simulink model "asm_basis_s"  (R2024a)
settings: Solver=ode45  StartTime=0.0  StopTime=0.5  FixedStep=Ta  MaxStep=1e-5  RelTol=1e-3  EnableMultiTasking=on
values from neighbouring files (symbols this model uses):
  ASM_Lh = 0.404    [init_asm_basis.m]
  ASM_Lr = ASM_Lrsigma + ASM_Lh    (= 0.41305)    [init_asm_basis.m]
  ASM_Ls = ASM_Lssigma + ASM_Lh    (= 0.41305)    [init_asm_basis.m]
  ASM_p = 1    [init_asm_basis.m]
  ASM_PSI_RN = 0.98    [init_asm_basis.m]
  ASM_Rr = 1.6    [init_asm_basis.m]
  ASM_sigma = 1-ASM_Lh^2/(ASM_Ls*ASM_Lr)    (= 0.0433403047275)    [init_asm_basis.m]
  CC_KAW = 1/ASM_TN    (= 303.359547356)    [init_asm_basis.m]
  CC_KI = CC_KP/ASM_T1    [init_asm_basis.m]
  CC_KP = (ASM_T1)/(2*ASM_K*ASM_Tsigma)    [init_asm_basis.m]
  f_sw = 5e3    (= 5000)    [init_asm_basis.m]
  FC_KAW = 1/FC_TN    (= 3.87362304806)    [init_asm_basis.m]
  FC_KI = FC_KP/FC_T1    [init_asm_basis.m]
  FC_KP = (FC_T1)/(2*FC_K*FC_Tsigma)    [init_asm_basis.m]
  imax = 6    [init_asm_basis.m]
  n_N = 2895    [init_asm_basis.m]
  SC_KAW = 1/(SC_a^2*SC_T_sigma)    [init_asm_basis.m]
  SC_KI = SC_KP/(SC_a^2*SC_T_sigma)    [init_asm_basis.m]
  SC_KP = SC_T1/(SC_a*SC_K*SC_T_sigma)    [init_asm_basis.m]
  Ta = 1/fa    (= 0.0002)    [init_asm_basis.m]
  udc = 400*sqrt(2)    [init_asm_basis.m]
  umax = udc/sqrt(3)    [init_asm_basis.m]
undefined symbols (not defined in the file or in its folder): DiscIntNeverNeededParam, plecs, sigbuilder_block
libraries: plecslib_extras2 x1, spsabctodq0Lib x1
settings Model: Creator=mabo  LastModifiedBy=mi
settings SolverCC: AlgebraicLoopSolver=TrustRegion
settings DataIOCC: LimitDataPoints=on  SaveFormat=Array  SignalLoggingSaveFormat=ModelDataLogs  ReturnWorkspaceOutputs=off
settings OptimizationCC: ExpressionDepthLimit=2147483647  LifeSpan=inf
settings DebuggingCC: UnderspecifiedInitializationDetection=Classic  MergeDetectMultiDrivingBlocksExec=none  SolverPrmCheckMsg=warning  FcnCallInpInsideContextMsg=warning  UnconnectedInputMsg=warning  UnconnectedOutputMsg=warning  UnconnectedLineMsg=warning  StateNameClashWarn=warning  SFUnexpectedBacktrackingDiag=warning  SFNoUnconditionalDefaultTransitionDiag=warning  SFExecutionAtInitializationDiag=none  ArithmeticOperatorsInVariantConditions=warning
settings HardwareCC: ProdBitPerPointer=32  ProdBitPerSizeT=32  ProdBitPerPtrDiffT=32  ProdLargestAtomicFloat=None  ProdIntDivRoundTo=Undefined  ProdEndianess=Unspecified  ProdWordSize=32  ProdHWDeviceType=32-bit Generic
settings ModelReferenceCC: EnableRefExpFcnMdlSchedulingChecks=on  PropagateSignalLabelsOutOfModel=off
settings SFSimCC: SimUseLocalCustomCode=off  SimParseCustomCode=off  CustomCodeUndefinedFunction=UseInterfaceOnly
settings RTWCC: RTWUseLocalCustomCode=off  GPUComputeCapability=3.5  DLArmComputeVersion=19.05
settings CodeAppCC: StateflowObjectComments=on
settings GRTTargetCC: TargetLangStandard=C89/C90 (ANSI)  CombineOutputUpdateFcns=off  GRTInterface=on
settings ConfigComp: CovMetricSettings=dw  CovSaveCumulativeToWorkspaceVar=on  CovSaveSingleToWorkspaceVar=on  CovExternalEMLEnable=off  CovSFcnEnable=off

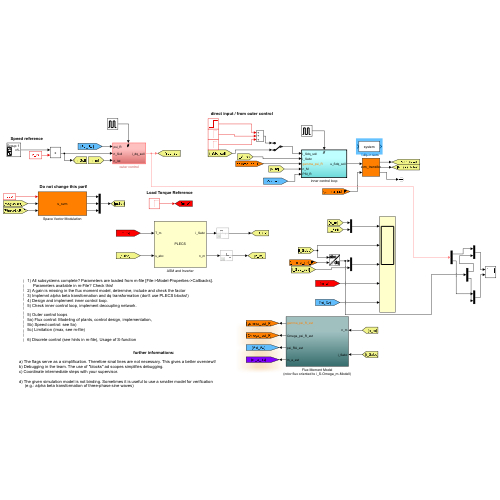
[thumbnail: Simulink's stored preview of the top-level diagram]
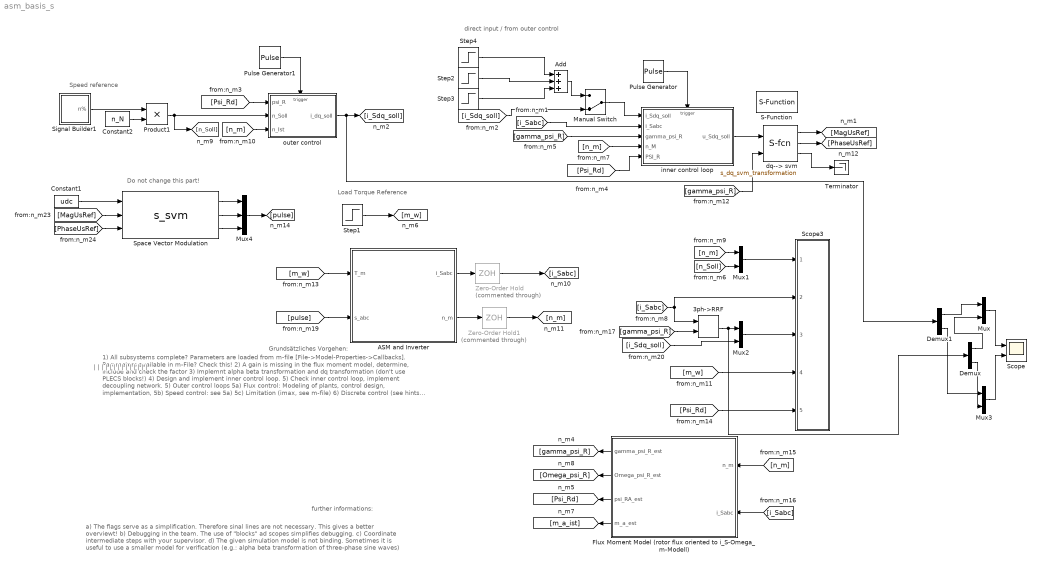
== system asm_basis_s ==
  note: Load Torque Reference
  note: Speed reference
  note: direct input / from outer control
  note: 1) All subsystems complete? Parameters are loaded from m-file [File->Model-Properties->Callbacks].
      |      Parameters available in m-File? Check this!
      | 2) A gain is missing in the flux moment model, determine, include and check the factor
      | 3) Implemnt alpha beta transformation and dq transformation (don't use PLECS blocks!)
      | 4) Design and implement inner control loop.
      | 5) Check inner control loop, implement decoupling network.
      |
      | 5) Outer control loops
      | 5a) Flux control: Modeling of plants, control design, implementation,
      | 5b) Speed control: see 5a)
      | 5c) Limitation (imax, see m-file)
      |
      | 6) Discrete control (see hints in m-file), Usage of S-function
  note: |
      | |
      | |
      | |
      | |
      | |
      | |
      | |
      | |
      | |
      | |
      | |
      | |
      | |
  note: Grundsätzliches Vorgehen:
  note: further informations:
  note: Do not change this part!
  note: a) The flags serve as a simplification. Therefore sinal lines are not necessary. This gives a better overviewt!
      | b) Debugging in the team. The use of "blocks" ad scopes simplifies debugging.
      | c) Coordinate intermediate steps with your supervisor.
      |
      | d) The given simulation model is not binding. Sometimes it is useful to use a smaller model for verification
      |      (e.g.: alpha beta transformation of three-phase sine waves)
  3ph->RRF : plecslib_extras2/Transformations/3ph->RRF
      settings: SourceProductName=PLECS Extras
  ASM and Inverter : Subsystem  LoadFcn=plecs('sl', 200);  InitFcn=plecs('sl', 214);  StartFcn=plecs('sl', 208);  StopFcn=plecs('sl', 209);  mask(PlecsCircuit){PLECSData=<binary blob, 7640 chars, not shown>}
      mask prompts: PLECSData "PLECS Data (Do not delete or modify!)"
      mask help: Drag this block into a Simulink model to create a new electrical circuit.
      mask init:
      | % PLACE CUSTOM INITIALIZATIONS ABOVE
      | % DO NOT REMOVE
      | plecs('sl', 215);
      | % DO NOT REMOVE
      settings: CopyFcn=plecs('sl', 203);  DeleteFcn=plecs('sl', 205);  UndoDeleteFcn=plecs('sl', 206);  PreSaveFcn=plecs('sl', 211);  PostSaveFcn=plecs('sl', 201);  NameChangeFcn=plecs('sl', 210);  DestroyFcn=plecs('sl', 207);  PreCopyFcn=plecs('sl', 216);  OpenFcn=plecs('sl', 202);  ErrorFcn=plerrorfcn
      mask Display: disp('PLECS')
  Add : Sum  Inputs=+++
  Constant1 : Constant  Value=udc
  Constant2 : Constant  Value=n_N
  Demux : Demux  Outputs=2
  Demux1 : Demux  Outputs=2
  Flux Moment Model (rotor flux oriented to i_S-Omega_m-Modell) : Subsystem
  Manual Switch : ManualSwitch  CurrentSetting=0
  Mux{,1..3} (4 alike) : Mux  Inputs=2
  Mux4 : Mux  Inputs=3
  Product1 : Product  RndMeth=Zero
  Pulse Generator : DiscretePulseGenerator  PulseType=Time based  Period=Ta  PulseWidth=5
  Pulse Generator1 : DiscretePulseGenerator  PulseType=Time based  Period=Ta  PulseWidth=5
  S-Function : S-Function  SFunctionDeploymentMode=off  EnableBusSupport=off
  Scope : Scope  NumInputPorts=2
  Scope3 : Subsystem  LoadFcn=plecs('sl', 300);  InitFcn=plecs('sl', 314);  StartFcn=plecs('sl', 308);  StopFcn=plecs('sl', 309);  mask{Settings=<binary blob, 2020 chars, not shown>}
      mask init:
      | plecsedit('sl', 315);
      settings: CopyFcn=plecs('sl', 303);  DeleteFcn=plecs('sl', 305);  UndoDeleteFcn=plecs('sl', 306);  PreSaveFcn=plecs('sl', 311);  NameChangeFcn=plecs('sl', 310);  DestroyFcn=plecs('sl', 307);  OpenFcn=plecs('sl', 302);  ErrorFcn=plerrorfcn
      mask Display: plot([0.1 0.9 0.9 0.1 0.1], [0.9 0.9 0.5 0.5 0.9])
  Signal Builder1 : Subsystem  Tag=STV Subsys  LoadFcn=sigbuilder_block('load');  StartFcn=sigbuilder_block('start');  StopFcn=sigbuilder_block('stop');  ClipboardFcn=sigbuilder_block('clipboard');  mask(Sigbuilder block){tuvar=[0:10]}
      mask help: Sigbuilder GUI
      mask init:
      | if ~strcmp(get_param(bdroot(gcbh),'SimulationStatus'),'stopped') tuvar = sigbuilder_block('maskInit'); end
      settings: CopyFcn=sigbuilder_block('copy');  DeleteFcn=sigbuilder_block('delete');  ModelCloseFcn=sigbuilder_block('modelClose');  PreSaveFcn=sigbuilder_block('preSave');  PauseFcn=sigbuilder_block('pause')  ContinueFcn=sigbuilder_block('continue')  NameChangeFcn=sigbuilder_block('namechange');  OpenFcn=sigbuilder_block('open',[29.25 172.2 550.5 395.55 ]);  CloseFcn=sigbuilder_block('close');
      mask Display: plot(0, 0, 100, 100,[2, 2, 32, 32, 2], [68, 8, 8, 68, 68],[32, 2], [38, 38], [32, 19, 2],[53, 60, 44], [32, 17, 17, 2],[16, 16, 31, 31]);txt = getActiveGroup(gcbh);text(2, 100, txt,'verticalAlignment', 'top');
  Space Vector Modulation : S-Function  FunctionName=s_svm  Parameters=f_sw*100,f_sw  SFunctionDeploymentMode=off  EnableBusSupport=off
  Step1 : Step  Time=9  After=2  SampleTime=0
  Step2 : Step  Time=0.1  Before=[1.5 0]  After=[1.5 2]  SampleTime=0
  Step3 : Step  Time=0.2  Before=[0 0]  After=[0 -2]  SampleTime=0
  Step4 : Step  Time=0.05  Before=[-1.5 0]  After=[0 0]  SampleTime=0
  Terminator : Terminator
  Zero-Order Hold : ZeroOrderHold  Commented=through  SampleTime=Ta
  Zero-Order Hold1 : ZeroOrderHold  Commented=through  SampleTime=Ta
  dq--> svm : S-Function  FunctionName=s_dq_svm_transformation  Parameters=f_sw  SFunctionDeploymentMode=off  EnableBusSupport=off
  inner control loop : Subsystem
  outer control : Subsystem
  wires:
  outer control/1(i_dq_soll) -> Demux1/1, [i_Sdq_soll]
  Step1/1 -> [m_w]
  [i_Sabc] -> inner control loop/2(i_Sabc)
  [i_Sdq_soll] -> Manual Switch/2
  [gamma_psi_R] -> inner control loop/3(gamma_psi_R)
  [n_m] -> outer control/3(n_Ist)
  Constant2/1 -> Product1/2
  Signal Builder1/1(n%) -> Product1/1
  Product1/1 -> [n_Soll], outer control/2(n_Soll)
  [m_w] -> ASM and Inverter/1(T_m)
  [pulse] -> ASM and Inverter/2(s_abc)
  Manual Switch/1 -> inner control loop/1(i_Sdq_soll)
  [Psi_Rd] -> outer control/1(psi_R)
  [Psi_Rd] -> inner control loop/5(PSI_R)
  [n_m] -> inner control loop/4(n_M)
  Add/1 -> Manual Switch/1
  Step2/1 -> Add/2
  Step3/1 -> Add/3
  Step4/1 -> Add/1
  ASM and Inverter/2(n_m) -> Zero-Order Hold1/1
  [n_m] -> Mux1/1
  [n_Soll] -> Mux1/2
  Mux1/1 -> Scope3/1(1)
  [i_Sabc] -> 3ph->RRF/1, Scope3/2(2)
  [gamma_psi_R] -> 3ph->RRF/2
  3ph->RRF/1 -> Demux/1, Mux2/1
  Mux2/1 -> Scope3/3(3)
  [m_w] -> Scope3/4(4)
  [Psi_Rd] -> Scope3/5(5)
  [PhaseUsRef] -> Space Vector Modulation/3
  [MagUsRef] -> Space Vector Modulation/2
  Constant1/1 -> Space Vector Modulation/1
  Space Vector Modulation/1 -> Mux4/1
  Space Vector Modulation/2 -> Mux4/2
  Space Vector Modulation/3 -> Mux4/3
  Mux4/1 -> [pulse]
  dq--> svm/1 -> [MagUsRef]
  dq--> svm/2 -> [PhaseUsRef]
  [gamma_psi_R] -> dq--> svm/2
  inner control loop/1(u_Sdq_soll) -> dq--> svm/1
  dq--> svm/3 -> Terminator/1
  [i_Sdq_soll] -> Mux2/2
  Flux Moment Model (rotor flux oriented to i_S-Omega_m-Modell)/1(gamma_psi_R_est) -> [gamma_psi_R]
  Flux Moment Model (rotor flux oriented to i_S-Omega_m-Modell)/4(m_a_est) -> [m_a_ist]
  [n_m] -> Flux Moment Model (rotor flux oriented to i_S-Omega_m-Modell)/1(n_m)
  [i_Sabc] -> Flux Moment Model (rotor flux oriented to i_S-Omega_m-Modell)/2(i_Sabc)
  Flux Moment Model (rotor flux oriented to i_S-Omega_m-Modell)/3(psi_RA_est) -> [Psi_Rd]
  Flux Moment Model (rotor flux oriented to i_S-Omega_m-Modell)/2(Omega_psi_R_est) -> [Omega_psi_R]
  Demux/1 -> Mux/2
  Demux1/1 -> Mux/1
  Mux/1 -> Scope/1
  Mux3/1 -> Scope/2
  Demux1/2 -> Mux3/1
  Demux/2 -> Mux3/2
  ASM and Inverter/1(i_Sabc) -> Zero-Order Hold/1
  Zero-Order Hold/1 -> [i_Sabc]
  Zero-Order Hold1/1 -> [n_m]
  Pulse Generator/1 -> inner control loop/Trigger
  Pulse Generator1/1 -> outer control/Trigger

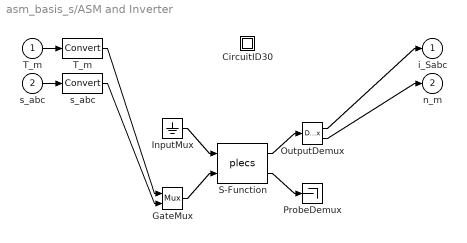
== system asm_basis_s/ASM and Inverter ==
  T_m : Inport  PortDimensions=1
  s_abc : Inport  Port=2  PortDimensions=3
  " CircuitID30 " : Subsystem
  " GateMux " : Mux  Inputs=[ 1 3 ]
  " InputMux " : Ground
  " OutputDemux " : Demux  Outputs=[ 3 1 ]
  " ProbeDemux " : Terminator
  " S-Function " : S-Function  FunctionName=plecs  SFunctionDeploymentMode=off  EnableBusSupport=off
  " T_m " : DataTypeConversion
  " s_abc " : DataTypeConversion
  i_Sabc : Outport  PortDimensions=3  VectorParamsAs1DForOutWhenUnconnected=off
  n_m : Outport  Port=2  PortDimensions=1  VectorParamsAs1DForOutWhenUnconnected=off
  wires:
  " InputMux "/1 -> " S-Function "/1
  " GateMux "/1 -> " S-Function "/2
  " S-Function "/1 -> " OutputDemux "/1
  " S-Function "/2 -> " ProbeDemux "/1
  T_m/1 -> " T_m "/1
  " T_m "/1 -> " GateMux "/1
  s_abc/1 -> " s_abc "/1
  " s_abc "/1 -> " GateMux "/2
  " OutputDemux "/1 -> i_Sabc/1
  " OutputDemux "/2 -> n_m/1

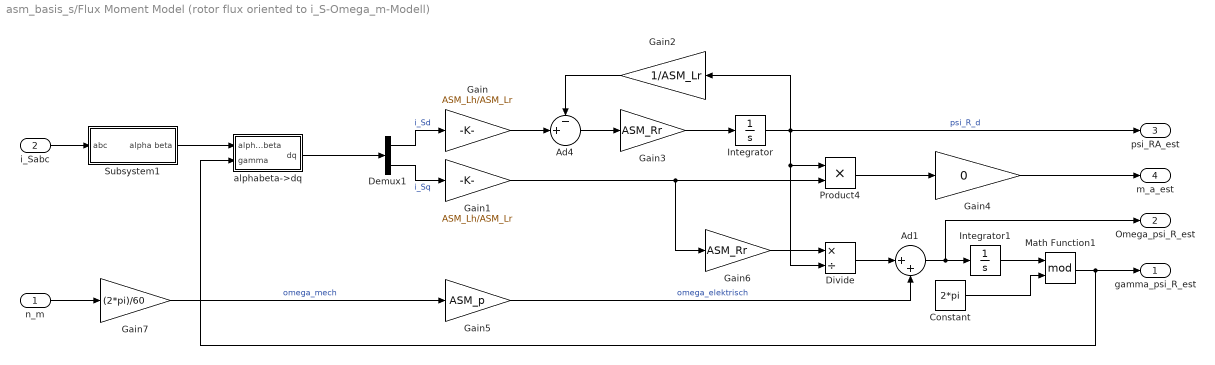
== system asm_basis_s/Flux Moment Model (rotor flux oriented to i_S-Omega_m-Modell) ==
  n_m : Inport
  i_Sabc : Inport  Port=2
  Ad1 : Sum  Inputs=|++
  Ad4 : Sum  Inputs=-+|
  Constant : Constant  Value=2*pi
  Demux1 : Demux  Outputs=2
  Divide : Product  Inputs=*/
  Gain : Gain  Gain=ASM_Lh/ASM_Lr
  Gain1 : Gain  Gain=ASM_Lh/ASM_Lr
  Gain2 : Gain  Gain=1/ASM_Lr
  Gain3 : Gain  Gain=ASM_Rr
  Gain4 : Gain  Gain=0
  Gain5 : Gain  Gain=ASM_p
  Gain6 : Gain  Gain=ASM_Rr
  Gain7 : Gain  Gain=(2*pi)/60
  Integrator : Integrator  InitialCondition=0.0001
  Integrator1 : Integrator  InitialCondition=0.0001
  Math Function1 : Math  Operator=mod  SignedPower=on
  Product4 : Product  RndMeth=Zero
  Subsystem1 : Subsystem
  alphabeta->dq : Subsystem
  gamma_psi_R_est : Outport  VectorParamsAs1DForOutWhenUnconnected=off
  Omega_psi_R_est : Outport  Port=2  VectorParamsAs1DForOutWhenUnconnected=off
  psi_RA_est : Outport  Port=3  VectorParamsAs1DForOutWhenUnconnected=off
  m_a_est : Outport  Port=4  VectorParamsAs1DForOutWhenUnconnected=off
  wires:
  Demux1/2 -> Gain1/1  "i_Sq"
  Demux1/1 -> Gain/1  "i_Sd"
  Gain/1 -> Ad4/2
  Ad4/1 -> Gain3/1
  Gain2/1 -> Ad4/1
  Gain3/1 -> Integrator/1
  Integrator/1 -> Gain2/1, psi_RA_est/1, Product4/1, Divide/2  "psi_R_d"
  Gain1/1 -> Product4/2, Gain6/1
  Product4/1 -> Gain4/1
  Gain4/1 -> m_a_est/1
  Divide/1 -> Ad1/1
  Ad1/1 -> Omega_psi_R_est/1, Integrator1/1
  Integrator1/1 -> Math Function1/1
  n_m/1 -> Gain7/1
  Gain5/1 -> Ad1/2  "omega_elektrisch"
  Math Function1/1 -> gamma_psi_R_est/1, alphabeta->dq/2(gamma)
  Gain6/1 -> Divide/1
  Subsystem1/1(alpha beta) -> alphabeta->dq/1(alphabeta)
  i_Sabc/1 -> Subsystem1/1(abc)
  alphabeta->dq/1(dq) -> Demux1/1
  Gain7/1 -> Gain5/1  "omega_mech"
  Constant/1 -> Math Function1/2

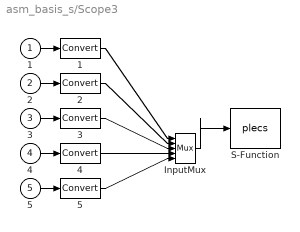
== system asm_basis_s/Scope3 ==
  1 : Inport
  2 : Inport  Port=2
  3 : Inport  Port=3
  4 : Inport  Port=4
  5 : Inport  Port=5
  " 1 " : DataTypeConversion
  " 2 " : DataTypeConversion
  " 3 " : DataTypeConversion
  " 4 " : DataTypeConversion
  " 5 " : DataTypeConversion
  " InputMux " : Mux  Inputs=5
  " S-Function " : S-Function  FunctionName=plecs  SFunctionDeploymentMode=off  EnableBusSupport=off
  wires:
  " InputMux "/1 -> " S-Function "/1
  1/1 -> " 1 "/1
  " 1 "/1 -> " InputMux "/1
  2/1 -> " 2 "/1
  " 2 "/1 -> " InputMux "/2
  3/1 -> " 3 "/1
  " 3 "/1 -> " InputMux "/3
  4/1 -> " 4 "/1
  " 4 "/1 -> " InputMux "/4
  5/1 -> " 5 "/1
  " 5 "/1 -> " InputMux "/5

== system asm_basis_s/Signal Builder1 ==
  Demux : Demux  Tag=STV Demux  Outputs=1
      settings: DisplayOption=none
  FromWs : FromWorkspace  Tag=STV FromWs  VariableName=tuvar
      SigBuilderData=|
      | common.afterFinalStr = 'Extrapolate'
      | common.sampleTime = 0
      | dataSet.timeRange = [0 1]
      | dataSet.name = 'Group 1'
      | sbobj.Groups.Name = 'Group 1'
      | sbobj.Groups.Signals.Name = 'n%'
      | sbobj.Groups.Signals.XData = [0 0.102 0.102 0.354 0.354 1]
      | sbobj.Groups.Signals.YData = [0 0 1 1 0.6 0.6]
      | sbobj.Groups.TimeRange = [0 1]
  n% : Outport  Tag=STV Outport  VectorParamsAs1DForOutWhenUnconnected=off
  wires:
  FromWs/1 -> Demux/1
  Demux/1 -> n%/1

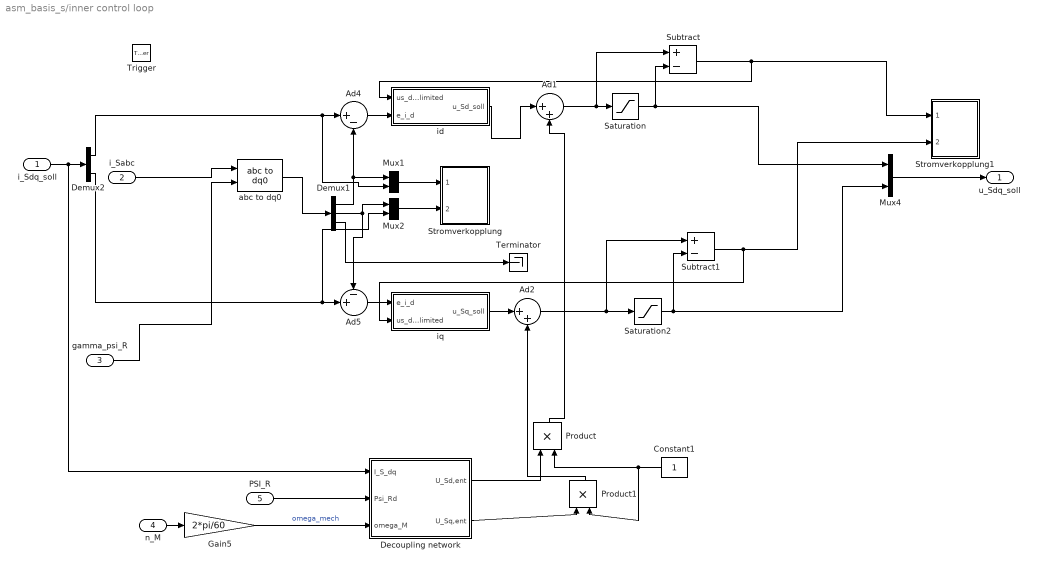
== system asm_basis_s/inner control loop ==
  i_Sdq_soll : Inport
  i_Sabc : Inport  Port=2
  gamma_psi_R : Inport  Port=3
  n_M : Inport  Port=4
  PSI_R : Inport  Port=5
  Trigger : TriggerPort  VariantControl=(inherit)  PortDimensions=1
  Ad1 : Sum  Inputs=|++
  Ad2 : Sum  Inputs=|++
  Ad4 : Sum  Inputs=|+-
  Ad5 : Sum  Inputs=-+|
  Constant1 : Constant
  Decoupling network : Subsystem
  Demux1 : Demux  Outputs=3
  Demux2 : Demux  Outputs=2
  Gain5 : Gain  Gain=2*pi/60
  Mux1 : Mux  Inputs=[1 1]
  Mux2 : Mux  Inputs=[1 1]
  Mux4 : Mux  Inputs=2
  Product : Product  RndMeth=Zero
  Product1 : Product  RndMeth=Zero
  Saturation : Saturate  UpperLimit=umax  LowerLimit=-umax
  Saturation2 : Saturate  UpperLimit=umax  LowerLimit=-umax
  Stromverkopplung : Subsystem  LoadFcn=plecs('sl', 300);  InitFcn=plecs('sl', 314);  StartFcn=plecs('sl', 308);  StopFcn=plecs('sl', 309);  mask{Settings=<binary blob, 1300 chars, not shown>}
      mask init:
      | plecsedit('sl', 315);
      settings: CopyFcn=plecs('sl', 303);  DeleteFcn=plecs('sl', 305);  UndoDeleteFcn=plecs('sl', 306);  PreSaveFcn=plecs('sl', 311);  NameChangeFcn=plecs('sl', 310);  DestroyFcn=plecs('sl', 307);  OpenFcn=plecs('sl', 302);  ErrorFcn=plerrorfcn
      mask Display: plot([0.1 0.9 0.9 0.1 0.1], [0.9 0.9 0.5 0.5 0.9])
  Stromverkopplung1 : Subsystem  LoadFcn=plecs('sl', 300);  InitFcn=plecs('sl', 314);  StartFcn=plecs('sl', 308);  StopFcn=plecs('sl', 309);  mask{Settings=<binary blob, 1192 chars, not shown>}
      mask init:
      | plecsedit('sl', 315);
      settings: CopyFcn=plecs('sl', 303);  DeleteFcn=plecs('sl', 305);  UndoDeleteFcn=plecs('sl', 306);  PreSaveFcn=plecs('sl', 311);  NameChangeFcn=plecs('sl', 310);  DestroyFcn=plecs('sl', 307);  OpenFcn=plecs('sl', 302);  ErrorFcn=plerrorfcn
      mask Display: plot([0.1 0.9 0.9 0.1 0.1], [0.9 0.9 0.5 0.5 0.9])
  Subtract : Sum  Inputs=+-
  Subtract1 : Sum  Inputs=+-
  Terminator : Terminator
  abc to dq0 : spsabctodq0Lib/abc to dq0  Alignment=Aligned with phase A axis
  id : Subsystem
  iq : Subsystem
  u_Sdq_soll : Outport  VectorParamsAs1DForOutWhenUnconnected=off
  wires:
  Ad4/1 -> id/2(e_i_d)
  Demux1/1 -> Ad4/2, Mux1/1
  Demux2/1 -> Ad4/1, Mux1/2
  Demux1/2 -> Ad5/1, Mux2/1
  Demux2/2 -> Mux2/2, Ad5/2
  Ad5/1 -> iq/1(e_i_d)
  i_Sdq_soll/1 -> Demux2/1, Decoupling network/1(I_S_dq)
  Mux1/1 -> Stromverkopplung/1(1)
  Mux2/1 -> Stromverkopplung/2(2)
  PSI_R/1 -> Decoupling network/2(Psi_Rd)
  n_M/1 -> Gain5/1
  Gain5/1 -> Decoupling network/3(omega_M)  "omega_mech"
  Decoupling network/2(U_Sq,ent) -> Product1/1
  Mux4/1 -> u_Sdq_soll/1
  Subtract1/1 -> iq/2(us_delta_limited), Stromverkopplung1/2(2)
  Constant1/1 -> Product/2, Product1/2
  Decoupling network/1(U_Sd,ent) -> Product/1
  Product/1 -> Ad1/2
  Product1/1 -> Ad2/2
  Demux1/3 -> Terminator/1
  Subtract/1 -> id/1(us_delta_limited), Stromverkopplung1/1(1)
  abc to dq0/1 -> Demux1/1
  Saturation/1 -> Mux4/1, Subtract/2
  id/1(u_Sd_soll) -> Ad1/1
  Saturation2/1 -> Mux4/2, Subtract1/2
  iq/1(u_Sq_soll) -> Ad2/1
  Ad1/1 -> Subtract/1, Saturation/1
  Ad2/1 -> Subtract1/1, Saturation2/1
  i_Sabc/1 -> abc to dq0/1
  gamma_psi_R/1 -> abc to dq0/2

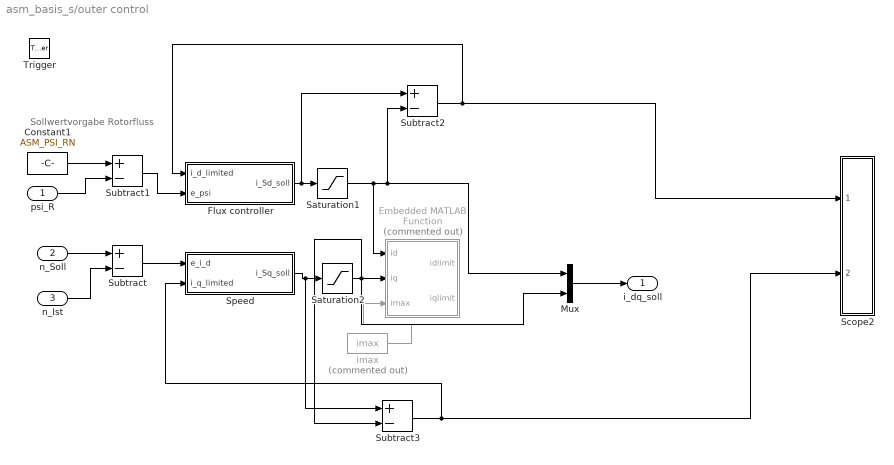
== system asm_basis_s/outer control ==
  note: Sollwertvorgabe
      |  Rotorfluss
  psi_R : Inport
  n_Soll : Inport  Port=2
  n_Ist : Inport  Port=3
  Trigger : TriggerPort  VariantControl=(inherit)  PortDimensions=1
  Constant1 : Constant  Value=ASM_PSI_RN
  Embedded MATLAB Function : MATLAB Function  Commented=on  TreatAsAtomicUnit=on
  Flux controller : Subsystem
  Mux : Mux  Inputs=[1 1]
  Saturation1 : Saturate  UpperLimit=imax  LowerLimit=-imax
  Saturation2 : Saturate  UpperLimit=imax  LowerLimit=-imax
  Scope2 : Subsystem  LoadFcn=plecs('sl', 300);  InitFcn=plecs('sl', 314);  StartFcn=plecs('sl', 308);  StopFcn=plecs('sl', 309);  mask{Settings=<binary blob, 1192 chars, not shown>}
      mask init:
      | plecsedit('sl', 315);
      settings: CopyFcn=plecs('sl', 303);  DeleteFcn=plecs('sl', 305);  UndoDeleteFcn=plecs('sl', 306);  PreSaveFcn=plecs('sl', 311);  NameChangeFcn=plecs('sl', 310);  DestroyFcn=plecs('sl', 307);  OpenFcn=plecs('sl', 302);  ErrorFcn=plerrorfcn
      mask Display: plot([0.1 0.9 0.9 0.1 0.1], [0.9 0.9 0.5 0.5 0.9])
  Speed : Subsystem
  Subtract{,1..3} (4 alike) : Sum  Inputs=+-
  imax : Constant  Commented=on  Value=imax
  i_dq_soll : Outport  InitialOutput=[0 0]  VectorParamsAs1DForOutWhenUnconnected=off
  wires:
  Flux controller/1(i_Sd_soll) -> Subtract2/1, Saturation1/1
  Speed/1(i_Sq_soll) -> Subtract3/1, Saturation2/1
  imax/1 -> Embedded MATLAB Function/3(imax)
  n_Soll/1 -> Subtract/1
  n_Ist/1 -> Subtract/2
  Subtract/1 -> Speed/1(e_i_d)
  Constant1/1 -> Subtract1/1
  psi_R/1 -> Subtract1/2
  Subtract1/1 -> Flux controller/2(e_psi)
  Mux/1 -> i_dq_soll/1
  Saturation1/1 -> Subtract2/2, Mux/1, Embedded MATLAB Function/1(id)
  Saturation2/1 -> Mux/2, Subtract3/2, Embedded MATLAB Function/2(iq)
  Subtract2/1 -> Flux controller/1(i_d_limited), Scope2/1(1)
  Subtract3/1 -> Speed/2(i_q_limited), Scope2/2(2)

== system asm_basis_s/ASM and Inverter/ CircuitID30  ==

== system asm_basis_s/Flux Moment Model (rotor flux oriented to i_S-Omega_m-Modell)/Subsystem1 ==
  note: Amplitudeninvariant
  abc : Inport  PortDimensions=3
  Mux : Mux  Inputs=2
  alpha : Fcn  Expr=(2*u(1)-u(2)-u(3))/3
  beta : Fcn  Expr=(u(2)-u(3))/sqrt(3)
  alpha beta : Outport  VectorParamsAs1DForOutWhenUnconnected=off
  wires:
  alpha/1 -> Mux/1
  beta/1 -> Mux/2
  abc/1 -> beta/1, alpha/1
  Mux/1 -> alpha beta/1

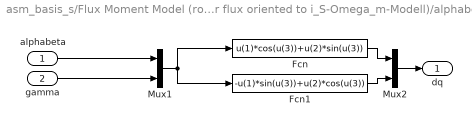
== system asm_basis_s/Flux Moment Model (rotor flux oriented to i_S-Omega_m-Modell)/alphabeta->dq ==
  alphabeta : Inport
  gamma : Inport  Port=2
  Fcn : Fcn  Expr=u(1)*cos(u(3))+u(2)*sin(u(3))
  Fcn1 : Fcn  Expr=-u(1)*sin(u(3))+u(2)*cos(u(3))
  Mux1 : Mux  Inputs=2
  Mux2 : Mux  Inputs=2
  dq : Outport  VectorParamsAs1DForOutWhenUnconnected=off
  wires:
  Mux2/1 -> dq/1
  Mux1/1 -> Fcn1/1, Fcn/1
  Fcn1/1 -> Mux2/2
  Fcn/1 -> Mux2/1
  alphabeta/1 -> Mux1/1
  gamma/1 -> Mux1/2

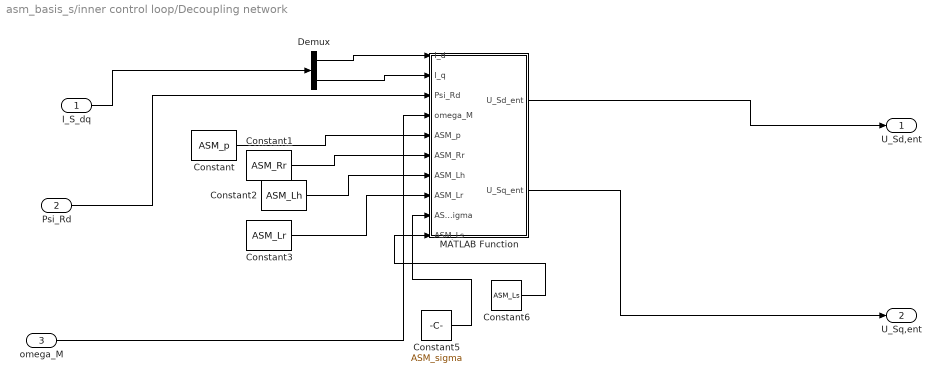
== system asm_basis_s/inner control loop/Decoupling network ==
  I_S_dq : Inport
  Psi_Rd : Inport  Port=2
  omega_M : Inport  Port=3
  Constant : Constant  Value=ASM_p
  Constant1 : Constant  Value=ASM_Rr
  Constant2 : Constant  Value=ASM_Lh
  Constant3 : Constant  Value=ASM_Lr
  Constant5 : Constant  Value=ASM_sigma
  Constant6 : Constant  Value=ASM_Ls
  Demux : Demux  Outputs=2
  MATLAB Function : MATLAB Function  TreatAsAtomicUnit=on
  U_Sd,ent : Outport  VectorParamsAs1DForOutWhenUnconnected=off
  U_Sq,ent : Outport  Port=2  VectorParamsAs1DForOutWhenUnconnected=off
  wires:
  I_S_dq/1 -> Demux/1
  Psi_Rd/1 -> MATLAB Function/3(Psi_Rd)
  omega_M/1 -> MATLAB Function/4(omega_M)
  MATLAB Function/1(U_Sd_ent) -> U_Sd,ent/1
  MATLAB Function/2(U_Sq_ent) -> U_Sq,ent/1
  Constant/1 -> MATLAB Function/5(ASM_p)
  Constant1/1 -> MATLAB Function/6(ASM_Rr)
  Constant2/1 -> MATLAB Function/7(ASM_Lh)
  Constant3/1 -> MATLAB Function/8(ASM_Lr)
  Demux/1 -> MATLAB Function/1(I_d)
  Demux/2 -> MATLAB Function/2(I_q)
  Constant5/1 -> MATLAB Function/9(ASM_sigma)
  Constant6/1 -> MATLAB Function/10(ASM_Ls)

== system asm_basis_s/inner control loop/Stromverkopplung ==
  1 : Inport
  2 : Inport  Port=2
  " InputMux " : Subsystem
      mask Display: disp('Mux')
  " S-Function " : S-Function  FunctionName=plecs  SFunctionDeploymentMode=off  EnableBusSupport=off
  wires:
  2/1 -> " InputMux "/2(In2)
  1/1 -> " InputMux "/1(In1)
  " InputMux "/1(Out) -> " S-Function "/1

== system asm_basis_s/inner control loop/Stromverkopplung1 ==
  1 : Inport
  2 : Inport  Port=2
  " InputMux " : Subsystem
      mask Display: disp('Mux')
  " S-Function " : S-Function  FunctionName=plecs  SFunctionDeploymentMode=off  EnableBusSupport=off
  wires:
  " InputMux "/1(Out) -> " S-Function "/1
  1/1 -> " InputMux "/1(In1)
  2/1 -> " InputMux "/2(In2)

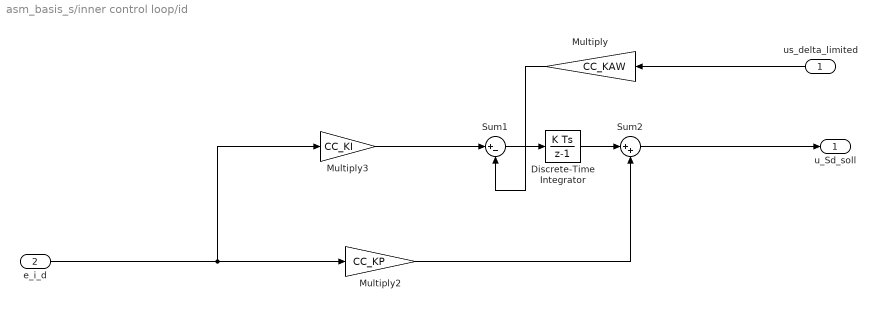
== system asm_basis_s/inner control loop/id ==
  us_delta_limited : Inport
  e_i_d : Inport  Port=2
  Discrete-Time Integrator : DiscreteIntegrator  SampleTime=-1  ICPrevOutput=DiscIntNeverNeededParam  ICPrevScaledInput=DiscIntNeverNeededParam
  Multiply : Gain  Gain=CC_KAW
  Multiply2 : Gain  Gain=CC_KP
  Multiply3 : Gain  Gain=CC_KI
  Sum1 : Sum  Inputs=|+-
  Sum2 : Sum  Inputs=|++
  u_Sd_soll : Outport  VectorParamsAs1DForOutWhenUnconnected=off
  wires:
  Multiply3/1 -> Sum1/1
  Sum1/1 -> Discrete-Time Integrator/1
  Multiply/1 -> Sum1/2
  Sum2/1 -> u_Sd_soll/1
  Multiply2/1 -> Sum2/2
  Discrete-Time Integrator/1 -> Sum2/1
  us_delta_limited/1 -> Multiply/1
  e_i_d/1 -> Multiply3/1, Multiply2/1

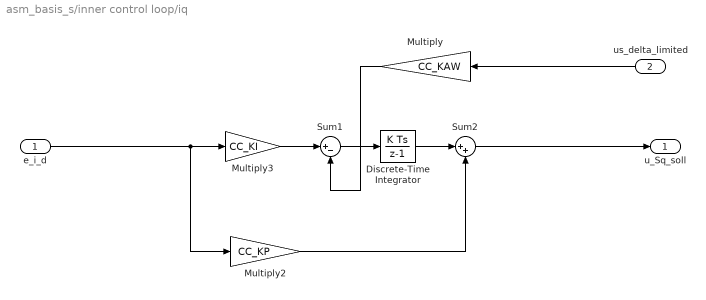
== system asm_basis_s/inner control loop/iq ==
  e_i_d : Inport
  us_delta_limited : Inport  Port=2
  Discrete-Time Integrator : DiscreteIntegrator  SampleTime=-1  ICPrevOutput=DiscIntNeverNeededParam  ICPrevScaledInput=DiscIntNeverNeededParam
  Multiply : Gain  Gain=CC_KAW
  Multiply2 : Gain  Gain=CC_KP
  Multiply3 : Gain  Gain=CC_KI
  Sum1 : Sum  Inputs=|+-
  Sum2 : Sum  Inputs=|++
  u_Sq_soll : Outport  VectorParamsAs1DForOutWhenUnconnected=off
  wires:
  Sum1/1 -> Discrete-Time Integrator/1
  Multiply/1 -> Sum1/2
  Multiply3/1 -> Sum1/1
  Discrete-Time Integrator/1 -> Sum2/1
  Multiply2/1 -> Sum2/2
  Sum2/1 -> u_Sq_soll/1
  e_i_d/1 -> Multiply2/1, Multiply3/1
  us_delta_limited/1 -> Multiply/1

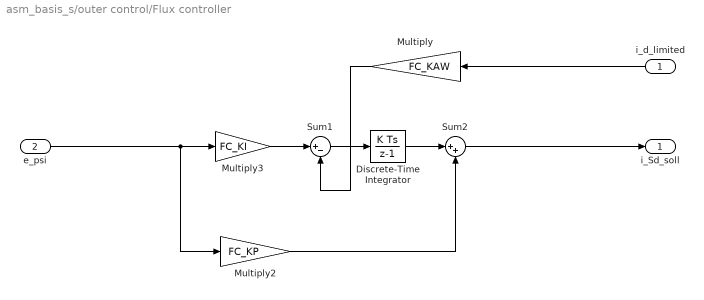
== system asm_basis_s/outer control/Flux controller ==
  i_d_limited : Inport
  e_psi : Inport  Port=2
  Discrete-Time Integrator : DiscreteIntegrator  SampleTime=-1  ICPrevOutput=DiscIntNeverNeededParam  ICPrevScaledInput=DiscIntNeverNeededParam
  Multiply : Gain  Gain=FC_KAW
  Multiply2 : Gain  Gain=FC_KP
  Multiply3 : Gain  Gain=FC_KI
  Sum1 : Sum  Inputs=|+-
  Sum2 : Sum  Inputs=|++
  i_Sd_soll : Outport  VectorParamsAs1DForOutWhenUnconnected=off
  wires:
  Sum1/1 -> Discrete-Time Integrator/1
  Multiply/1 -> Sum1/2
  i_d_limited/1 -> Multiply/1
  Multiply3/1 -> Sum1/1
  Discrete-Time Integrator/1 -> Sum2/1
  Multiply2/1 -> Sum2/2
  Sum2/1 -> i_Sd_soll/1
  e_psi/1 -> Multiply2/1, Multiply3/1

== system asm_basis_s/outer control/Scope2 ==
  1 : Inport
  2 : Inport  Port=2
  " InputMux " : Subsystem
      mask Display: disp('Mux')
  " S-Function " : S-Function  FunctionName=plecs  SFunctionDeploymentMode=off  EnableBusSupport=off
  wires:
  2/1 -> " InputMux "/2(In2)
  1/1 -> " InputMux "/1(In1)
  " InputMux "/1(Out) -> " S-Function "/1

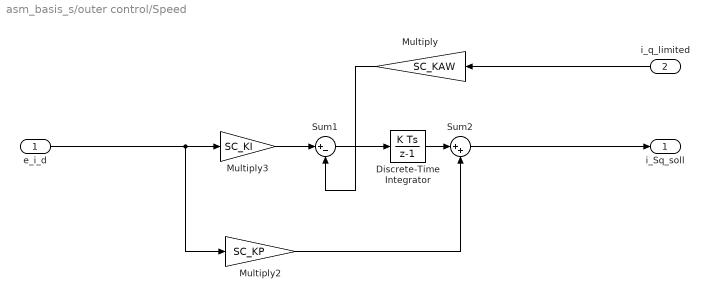
== system asm_basis_s/outer control/Speed ==
  e_i_d : Inport
  i_q_limited : Inport  Port=2
  Discrete-Time Integrator : DiscreteIntegrator  SampleTime=-1  ICPrevOutput=DiscIntNeverNeededParam  ICPrevScaledInput=DiscIntNeverNeededParam
  Multiply : Gain  Gain=SC_KAW
  Multiply2 : Gain  Gain=SC_KP
  Multiply3 : Gain  Gain=SC_KI
  Sum1 : Sum  Inputs=|+-
  Sum2 : Sum  Inputs=|++
  i_Sq_soll : Outport  VectorParamsAs1DForOutWhenUnconnected=off
  wires:
  Sum1/1 -> Discrete-Time Integrator/1
  Multiply2/1 -> Sum2/2
  Multiply3/1 -> Sum1/1
  Discrete-Time Integrator/1 -> Sum2/1
  Multiply/1 -> Sum1/2
  i_q_limited/1 -> Multiply/1
  e_i_d/1 -> Multiply2/1, Multiply3/1
  Sum2/1 -> i_Sq_soll/1

== system asm_basis_s/inner control loop/Stromverkopplung/ InputMux  ==
  In1 : Inport
  In2 : Inport  Port=2
  Convert1 : DataTypeConversion
  Convert2 : DataTypeConversion
  Mux : Mux  Inputs=2
  Out : Outport  VectorParamsAs1DForOutWhenUnconnected=off
  wires:
  Convert2/1 -> Mux/2
  Convert1/1 -> Mux/1
  In2/1 -> Convert2/1
  In1/1 -> Convert1/1
  Mux/1 -> Out/1

== system asm_basis_s/inner control loop/Stromverkopplung1/ InputMux  ==
  In1 : Inport
  In2 : Inport  Port=2
  Convert1 : DataTypeConversion
  Convert2 : DataTypeConversion
  Mux : Mux  Inputs=2
  Out : Outport  VectorParamsAs1DForOutWhenUnconnected=off
  wires:
  Mux/1 -> Out/1
  In1/1 -> Convert1/1
  In2/1 -> Convert2/1
  Convert1/1 -> Mux/1
  Convert2/1 -> Mux/2

== system asm_basis_s/outer control/Scope2/ InputMux  ==
  In1 : Inport
  In2 : Inport  Port=2
  Convert1 : DataTypeConversion
  Convert2 : DataTypeConversion
  Mux : Mux  Inputs=2
  Out : Outport  VectorParamsAs1DForOutWhenUnconnected=off
  wires:
  Convert2/1 -> Mux/2
  Convert1/1 -> Mux/1
  In2/1 -> Convert2/1
  In1/1 -> Convert1/1
  Mux/1 -> Out/1

== matlab function asm_basis_s/outer control/Embedded MATLAB Function ==
  data: id input; idlimit output; iq input; iqlimit output; imax input
function [idlimit,iqlimit] = fcn(id,iq,imax)
%#eml
idlimit=id;
iqlimit=iq;

== matlab function asm_basis_s/inner control loop/Decoupling network/MATLAB Function ==
  data: I_d input; I_q input; Psi_Rd input; omega_M input; U_Sd_ent output; U_Sq_ent output; ASM_p input; ASM_Rr input; ASM_Lh input; ASM_Lr input; ASM_sigma input; ASM_Ls input
function [U_Sd_ent,U_Sq_ent] = fcn(I_d,I_q, Psi_Rd, omega_M,ASM_p,ASM_Rr,ASM_Lh,ASM_Lr,ASM_sigma,ASM_Ls)
U_Sd_ent = ASM_sigma*ASM_Ls*(-ASM_p*omega_M*I_q-(ASM_Rr*ASM_Lh)/ASM_Lr/Psi_Rd*I_q^2)-Psi_Rd*ASM_Rr*ASM_Lh/ASM_Lr/ASM_Lr;
U_Sq_ent = ASM_sigma*ASM_Ls*(-ASM_p*omega_M*I_d+(ASM_Rr*ASM_Lh)/ASM_Lr/Psi_Rd*I_q*I_d)-ASM_p*omega_M*Psi_Rd*ASM_Lh/ASM_Lr;
